simulink model "HW7"  (R2024a)
settings: Solver=ode45  StartTime=0.0  StopTime=300  RelTol=1e-6  EnableMultiTasking=on
values from neighbouring files (symbols this model uses):
  A = [eye(3) -sqrt(3)/3*[1 1 1]' ]*Iwi    [set_up_HW7.m]    (also in setupConstantRateSDA.m)
  accelmax = 2/Iwi    (= 0.02)    [set_up_HW7.m]    (also in setupConstantRateSDA.m)
  c = Q(:,2)    [d2q.m]    (also in mbi.m = trace(Id)*.03; set_up_HW7.m = 0.001)
  I = [3000 0 0 ... (first row only)    [Constants_gui.m]    (also in constants.m; mbi.m = [15, .25, .20; set_up_HW7.m = I-Id; setupConstantRateSDA.m)
  Id = eye(3)*trace(I)*.003    [mbi.m]    (also in set_up_HW7.m = eye(3)*100)
  invI = inv(I)    [Constants_gui.m]    (also in constants.m; mbi.m; set_up_HW7.m; setupConstantRateSDA.m)
  invId = inv(Id)    [mbi.m]    (also in set_up_HW7.m)
  Kd = 2*zet*wn*I    [Constants_gui.m]    (also in constants.m = 2 * zet * wn * I; mbi.m = -eye(3)*.00002; set_up_HW7.m = 375000; setupConstantRateSDA.m)
  Kp = 2*wn^2*I    [Constants_gui.m]    (also in constants.m = 2 * wn^2 * I; mbi.m = -eye(3)*5.5; set_up_HW7.m = 300000; setupConstantRateSDA.m)
  pinvA = pinv(A)    [set_up_HW7.m]    (also in setupConstantRateSDA.m)
  q_init = q_init/norm(q_init)    [Constants_gui.m]    (also in constants.m = [-0.5 -0.5 -0.5 0.5]; mbi.m = [0 0 0 1]'; set_up_HW7.m = [0 0 0 1]'; setupConstantRateSDA.m)
  wbn_init = pi/30*[0 0 0]'    [Constants_gui.m]    (also in constants.m = pi/180 * [0.1; 0.2; 0.15]; mbi.m = [0 0 0]'; set_up_HW7.m = pi/30*[0 0 .01]'; setupConstantRateSDA.m)
  wdn_init = wbn_init    [mbi.m]    (also in set_up_HW7.m)
  wmax = 150/Iwi    (= 1.5)    [set_up_HW7.m]    (also in setupConstantRateSDA.m)
  ww0 = [0 0 0 0].'    [set_up_HW7.m]    (also in setupConstantRateSDA.m)
settings Model: Creator=Mason  LastModifiedBy=Spencer
settings SolverCC: AlgebraicLoopSolver=TrustRegion
settings DataIOCC: LimitDataPoints=on  SaveFormat=Array  SignalLoggingSaveFormat=ModelDataLogs  ReturnWorkspaceOutputs=off
settings OptimizationCC: ExpressionDepthLimit=2147483647  InitFltsAndDblsToZero=on  LifeSpan=inf
settings DebuggingCC: SaveWithParameterizedLinksMsg=none  UnderspecifiedInitializationDetection=Classic  MergeDetectMultiDrivingBlocksExec=none  SignalResolutionControl=TryResolveAllWithWarning  SolverPrmCheckMsg=warning  MultiTaskDSMMsg=warning  MultiTaskCondExecSysMsg=none  FcnCallInpInsideContextMsg=warning  UnconnectedInputMsg=warning  UnconnectedOutputMsg=warning  UnconnectedLineMsg=warning  StateNameClashWarn=warning  SFUnexpectedBacktrackingDiag=warning  SFNoUnconditionalDefaultTransitionDiag=warning  SFExecutionAtInitializationDiag=none  ArithmeticOperatorsInVariantConditions=warning
settings HardwareCC: ProdBitPerPointer=32  ProdBitPerSizeT=32  ProdBitPerPtrDiffT=32  ProdLargestAtomicFloat=None  ProdIntDivRoundTo=Undefined  ProdEndianess=Unspecified  ProdWordSize=32  ProdHWDeviceType=32-bit Generic
settings ModelReferenceCC: EnableRefExpFcnMdlSchedulingChecks=on  PropagateSignalLabelsOutOfModel=off
settings SFSimCC: SimUseLocalCustomCode=off  CustomCodeUndefinedFunction=UseInterfaceOnly
settings RTWCC: RTWUseLocalCustomCode=off  GPUComputeCapability=3.5  DLArmComputeVersion=19.05
settings CodeAppCC: StateflowObjectComments=on
settings GRTTargetCC: TargetFcnLib=ansi_tfl_tmw.mat  TargetLangStandard=C89/C90 (ANSI)  CombineOutputUpdateFcns=off  GRTInterface=on
settings ConfigComp: CovMetricSettings=dw  CovSaveCumulativeToWorkspaceVar=on  CovSaveSingleToWorkspaceVar=on  CovExternalEMLEnable=off

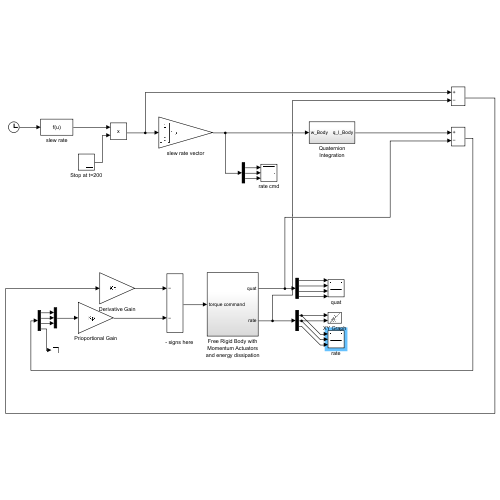
[thumbnail: Simulink's stored preview of the top-level diagram]
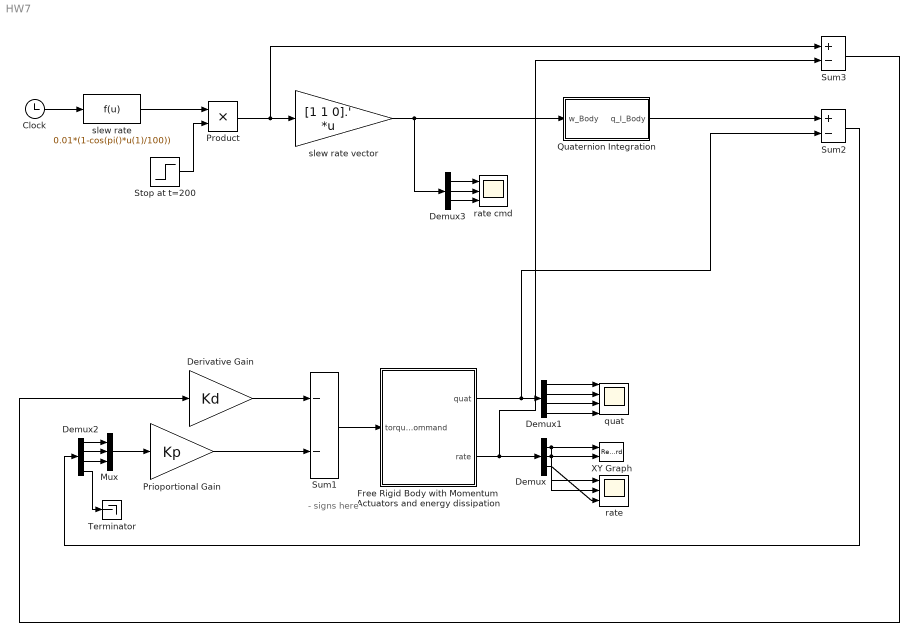
== system HW7 ==
  note: - signs here
  Clock : Clock
  Demux : Demux  Outputs=3
  Demux1 : Demux
  Demux2 : Demux
  Demux3 : Demux  Outputs=3
  Derivative Gain : Gain  Gain=Kd  SaturateOnIntegerOverflow=on  OutDataTypeStr=Inherit: Same as input  ParamDataTypeStr=Inherit: Same as input
  Free Rigid Body with Momentum Actuators and energy dissipation : Subsystem
  Mux : Mux  Inputs=3
  Prioportional Gain : Gain  Gain=Kp  SaturateOnIntegerOverflow=on  OutDataTypeStr=Inherit: Same as input  ParamDataTypeStr=Inherit: Same as input
  Product : Product  InputSameDT=on  SaturateOnIntegerOverflow=on  OutDataTypeStr=Inherit: Same as first input
  Quaternion Integration : Subsystem
  Stop at t=200 : Step  Time=200  Before=1  After=0  SampleTime=0
  Sum1 : Sum  Inputs=--  InputSameDT=on  SaturateOnIntegerOverflow=on  OutDataTypeStr=Inherit: Same as first input
  Sum2 : Sum  Inputs=+-  InputSameDT=on  SaturateOnIntegerOverflow=on  OutDataTypeStr=Inherit: Same as first input
  Sum3 : Sum  Inputs=+-  InputSameDT=on  SaturateOnIntegerOverflow=on  OutDataTypeStr=Inherit: Same as first input
  Terminator : Terminator
  XY Graph : Record  FileSettingsInternal="{\"entries\":[{\"content\":{\"excelSettings\":{\"content\":{},\"type\":\"Streamout.ExcelSettings\"}},\"type\":\"Streamout.FileSettingStorage\",\"uuid\":\"\"}],\"packageUris\":[\"http:\\/\\/schema.mathworks.com\\/mf0\\/streamout_blocks\\/R2020a\"],\"version\":\"1.0\"}"  Layout=[1 1]  SignalsInternal="{\"entries\":[{\"content\":{\"signals\":[{\"content\":{\"blockPath\":[],\"dimensions\":[1],\"domain\":\"\",\"lineColor\":\"#a2142f\",\"plots\":[ 1 ],\"port\":1,\"sid\":[\"\"],\"signalID\":1,\"signalName\":\"Demux:1\"},\"type\":\"RecordBlkView.Signal\",\"uuid\":\"\"},{\"content\":{\"blockPath\":[],\"dimensions\":[1],\"domain\":\"\",\"lineColor\":\"#139fff\",\"plots\":[ 1 ],\"port\":2,\"sid\":[\"\"],\"signalID\":2,\"signalName\":\"Demux:2\"},\"type\":\"RecordBlkView.Signal\",\"uuid\":\"\"}]},\"type\":\"RecordBlkView.InputSignals\",\"uuid\":\"\"}],\"packageUris\":[\"http:\\/\\/schema.mathworks.com\\/mf0\\/streamout_blocks\\/R2020a\"],\"version\":\"1.0\"}"  VisualizationBindings="{\"xyplotplugin\":{\"info\":[{\"series\":[{\"bindingParametersList\":[{\"parameter\":\"X-Axis\",\"signalID\":1,\"signalName\":\"Demux:1\"},{\"parameter\":\"Y-Axis\",\"signalID\":2,\"signalName\":\"Demux:2\"}],\"seriesID\":0}],\"subplotID\":1}]}}"  CompatibilityTag=XY  st=.25
  quat : Scope  NumInputPorts=4
  rate : Scope  NumInputPorts=3
  rate cmd : Scope  NumInputPorts=3
  slew rate : Fcn  Expr=0.01*(1-cos(pi()*u(1)/100))
  slew rate vector : Gain  Gain=[1 1 0].'  Multiplication=Matrix(K*u)  SaturateOnIntegerOverflow=on  OutDataTypeStr=Inherit: Same as input  ParamDataTypeStr=Inherit: Same as input
  wires:
  Demux1/1 -> quat/1
  Demux1/2 -> quat/2
  Demux1/3 -> quat/3
  Demux1/4 -> quat/4
  Demux/1 -> rate/1, XY Graph/1
  Demux/2 -> rate/2, XY Graph/2
  Demux/3 -> rate/3
  Free Rigid Body with Momentum Actuators and energy dissipation/2(rate) -> Sum3/2, Demux/1
  Free Rigid Body with Momentum Actuators and energy dissipation/1(quat) -> Sum2/2, Demux1/1
  Sum1/1 -> Free Rigid Body with Momentum Actuators and energy dissipation/1(torque command)
  Mux/1 -> Prioportional Gain/1
  Derivative Gain/1 -> Sum1/1
  Demux2/2 -> Mux/2
  Demux2/1 -> Mux/1
  Demux2/3 -> Mux/3
  Demux2/4 -> Terminator/1
  Prioportional Gain/1 -> Sum1/2
  Clock/1 -> slew rate/1
  slew rate vector/1 -> Quaternion Integration/1(w_Body), Demux3/1
  Quaternion Integration/1(q_I_Body) -> Sum2/1
  Sum2/1 -> Demux2/1
  Sum3/1 -> Derivative Gain/1
  slew rate/1 -> Product/1
  Stop at t=200/1 -> Product/2
  Product/1 -> Sum3/1, slew rate vector/1
  Demux3/1 -> rate cmd/1
  Demux3/2 -> rate cmd/2
  Demux3/3 -> rate cmd/3

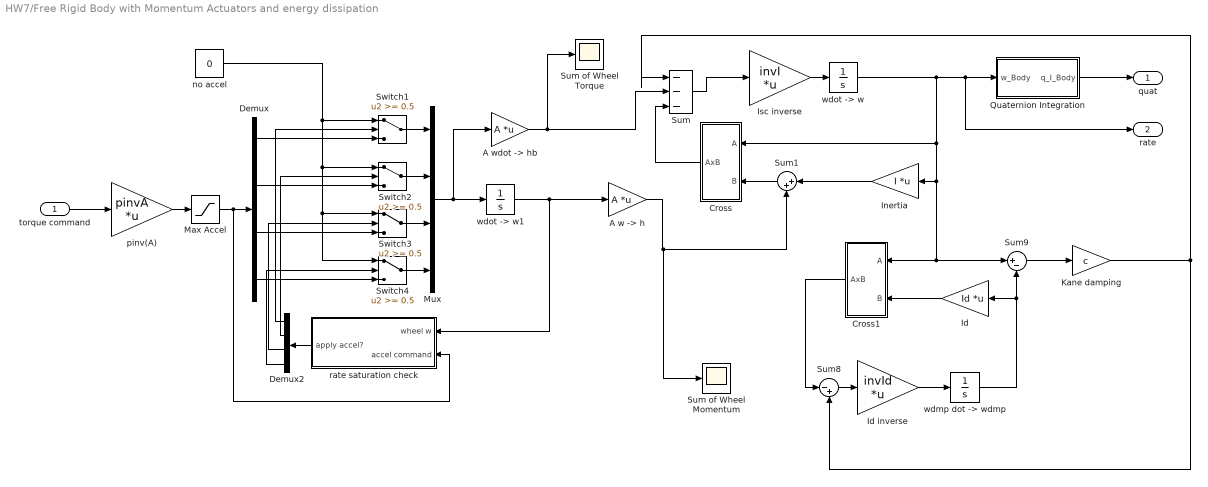
== system HW7/Free Rigid Body with Momentum Actuators and energy dissipation ==
  torque command : Inport
  "A w -> h" : Gain  Gain=A  Multiplication=Matrix(K*u)  SaturateOnIntegerOverflow=on  OutDataTypeStr=Inherit: Same as input  ParamDataTypeStr=Inherit: Same as input
  "A wdot -> hb" : Gain  Gain=A  Multiplication=Matrix(K*u)  SaturateOnIntegerOverflow=on  OutDataTypeStr=Inherit: Same as input  ParamDataTypeStr=Inherit: Same as input
  Cross : Subsystem
  Cross1 : Subsystem
  Demux : Demux
      settings: DisplayOption=none
  Demux2 : Demux
      settings: DisplayOption=none
  Id : Gain  Gain=Id  Multiplication=Matrix(K*u)  SaturateOnIntegerOverflow=on  OutDataTypeStr=Inherit: Same as input  ParamDataTypeStr=Inherit: Same as input
  Id inverse : Gain  Gain=invId  Multiplication=Matrix(K*u)  SaturateOnIntegerOverflow=on  OutDataTypeStr=Inherit: Same as input  ParamDataTypeStr=Inherit: Same as input
  Inertia : Gain  Gain=I  Multiplication=Matrix(K*u)  SaturateOnIntegerOverflow=on  OutDataTypeStr=Inherit: Same as input  ParamDataTypeStr=Inherit: Same as input
  Isc inverse : Gain  Gain=invI  Multiplication=Matrix(K*u)  SaturateOnIntegerOverflow=on  OutDataTypeStr=Inherit: Same as input  ParamDataTypeStr=Inherit: Same as input
  Kane damping : Gain  Gain=c  SaturateOnIntegerOverflow=on  OutDataTypeStr=Inherit: Same as input  ParamDataTypeStr=Inherit: Same as input
  Max Accel : Saturate  UpperLimit=accelmax  LowerLimit=-accelmax
  Mux : Mux
  Quaternion Integration : Subsystem
  Sum : Sum  Inputs=|---  InputSameDT=on  SaturateOnIntegerOverflow=on  OutDataTypeStr=Inherit: Same as first input
  Sum of Wheel Momentum : Scope
  Sum of Wheel Torque : Scope
  Sum1 : Sum  Inputs=|++  InputSameDT=on  SaturateOnIntegerOverflow=on  OutDataTypeStr=Inherit: Same as first input
  Sum8 : Sum  Inputs=|-+  InputSameDT=on  SaturateOnIntegerOverflow=on  OutDataTypeStr=Inherit: Same as first input
  Sum9 : Sum  Inputs=|+-  InputSameDT=on  SaturateOnIntegerOverflow=on  OutDataTypeStr=Inherit: Same as first input
  Switch{1..4} (4 alike) : Switch  Threshold=0.5
  no accel : Constant  Value=0
  pinv(A) : Gain  Gain=pinvA  Multiplication=Matrix(K*u)  SaturateOnIntegerOverflow=on  OutDataTypeStr=Inherit: Same as input  ParamDataTypeStr=Inherit: Same as input
  rate saturation check : Subsystem
  "wdmp dot -> wdmp" : Integrator  InitialCondition=wdn_init
  "wdot -> w" : Integrator  InitialCondition=wbn_init
  "wdot -> w1" : Integrator  InitialCondition=ww0
  quat : Outport
  rate : Outport  Port=2
  wires:
  Isc inverse/1 -> "wdot -> w"/1
  Sum9/1 -> Kane damping/1
  Sum8/1 -> Id inverse/1
  Id/1 -> Cross1/2(B)
  "wdmp dot -> wdmp"/1 -> Id/1, Sum9/2
  Id inverse/1 -> "wdmp dot -> wdmp"/1
  "wdot -> w"/1 -> rate/1, Quaternion Integration/1(w_Body), Sum9/1, Cross1/1(A), Inertia/1, Cross/1(A)
  Sum/1 -> Isc inverse/1
  Cross/1(AxB) -> Sum/3
  Max Accel/1 -> Demux/1, rate saturation check/2(accel command)
  Demux2/1 -> Switch1/2
  Demux2/3 -> Switch3/2
  no accel/1 -> Switch1/1, Switch4/1, Switch3/1, Switch2/1
  pinv(A)/1 -> Max Accel/1
  Demux2/4 -> Switch4/2
  "A wdot -> hb"/1 -> Sum of Wheel Torque/1, Sum/2
  "A w -> h"/1 -> Sum of Wheel Momentum/1, Sum1/2
  Inertia/1 -> Sum1/1
  Sum1/1 -> Cross/2(B)
  Mux/1 -> "wdot -> w1"/1, "A wdot -> hb"/1
  torque command/1 -> pinv(A)/1
  "wdot -> w1"/1 -> "A w -> h"/1, rate saturation check/1(wheel w)
  Quaternion Integration/1(q_I_Body) -> quat/1
  Kane damping/1 -> Sum8/2, Sum/1
  Cross1/1(AxB) -> Sum8/1
  Switch1/1 -> Mux/1
  Switch2/1 -> Mux/2
  Switch3/1 -> Mux/3
  Switch4/1 -> Mux/4
  Demux/1 -> Switch1/3
  Demux/2 -> Switch2/3
  Demux/3 -> Switch3/3
  Demux/4 -> Switch4/3
  rate saturation check/1(apply accel?) -> Demux2/1
  Demux2/2 -> Switch2/2

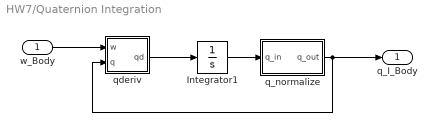
== system HW7/Quaternion Integration ==
  w_Body : Inport
  Integrator1 : Integrator  InitialCondition=q_init
  q_normalize : Subsystem
  qderiv : Subsystem
  q_I_Body : Outport
  wires:
  w_Body/1 -> qderiv/1(w)
  q_normalize/1(q_out) -> qderiv/2(q), q_I_Body/1
  Integrator1/1 -> q_normalize/1(q_in)
  qderiv/1(qd) -> Integrator1/1

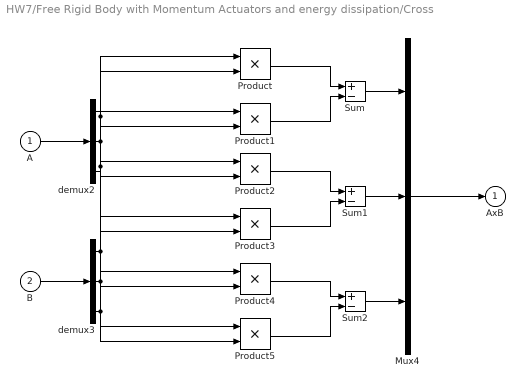
== system HW7/Free Rigid Body with Momentum Actuators and energy dissipation/Cross ==
  A : Inport
  B : Inport  Port=2
  Mux4 : Mux  Inputs=3
  Product{,1..5} (6 alike) : Product  InputSameDT=on  SaturateOnIntegerOverflow=on  OutDataTypeStr=Inherit: Same as first input
  Sum : Sum  Inputs=+-  InputSameDT=on  SaturateOnIntegerOverflow=on  OutDataTypeStr=Inherit: Same as first input
  Sum1 : Sum  Inputs=+-  InputSameDT=on  SaturateOnIntegerOverflow=on  OutDataTypeStr=Inherit: Same as first input
  Sum2 : Sum  Inputs=+-  InputSameDT=on  SaturateOnIntegerOverflow=on  OutDataTypeStr=Inherit: Same as first input
  demux2 : Demux  Outputs=3
      settings: DisplayOption=none
  demux3 : Demux  Outputs=3
      settings: DisplayOption=none
  AxB : Outport  InitialOutput=0
  wires:
  A/1 -> demux2/1
  B/1 -> demux3/1
  demux2/3 -> Product1/1, Product2/1
  demux3/3 -> Product/2, Product3/2
  demux2/1 -> Product3/1, Product4/1
  demux3/2 -> Product1/2, Product4/2
  demux2/2 -> Product/1, Product5/1
  demux3/1 -> Product2/2, Product5/2
  Product/1 -> Sum/1
  Product1/1 -> Sum/2
  Product2/1 -> Sum1/1
  Product3/1 -> Sum1/2
  Product4/1 -> Sum2/1
  Product5/1 -> Sum2/2
  Sum/1 -> Mux4/1
  Sum1/1 -> Mux4/2
  Sum2/1 -> Mux4/3
  Mux4/1 -> AxB/1

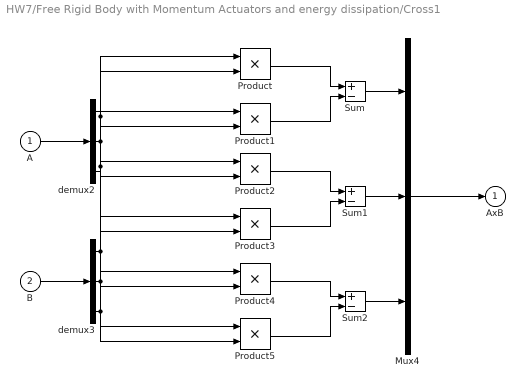
== system HW7/Free Rigid Body with Momentum Actuators and energy dissipation/Cross1 ==
  A : Inport
  B : Inport  Port=2
  Mux4 : Mux  Inputs=3
  Product{,1..5} (6 alike) : Product  InputSameDT=on  SaturateOnIntegerOverflow=on  OutDataTypeStr=Inherit: Same as first input
  Sum : Sum  Inputs=+-  InputSameDT=on  SaturateOnIntegerOverflow=on  OutDataTypeStr=Inherit: Same as first input
  Sum1 : Sum  Inputs=+-  InputSameDT=on  SaturateOnIntegerOverflow=on  OutDataTypeStr=Inherit: Same as first input
  Sum2 : Sum  Inputs=+-  InputSameDT=on  SaturateOnIntegerOverflow=on  OutDataTypeStr=Inherit: Same as first input
  demux2 : Demux  Outputs=3
      settings: DisplayOption=none
  demux3 : Demux  Outputs=3
      settings: DisplayOption=none
  AxB : Outport  InitialOutput=0
  wires:
  A/1 -> demux2/1
  B/1 -> demux3/1
  demux2/3 -> Product1/1, Product2/1
  demux3/3 -> Product/2, Product3/2
  demux2/1 -> Product3/1, Product4/1
  demux3/2 -> Product1/2, Product4/2
  demux2/2 -> Product/1, Product5/1
  demux3/1 -> Product2/2, Product5/2
  Product/1 -> Sum/1
  Product1/1 -> Sum/2
  Product2/1 -> Sum1/1
  Product3/1 -> Sum1/2
  Product4/1 -> Sum2/1
  Product5/1 -> Sum2/2
  Sum/1 -> Mux4/1
  Sum1/1 -> Mux4/2
  Sum2/1 -> Mux4/3
  Mux4/1 -> AxB/1

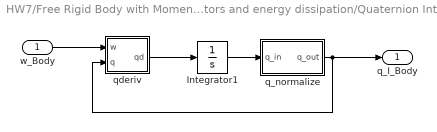
== system HW7/Free Rigid Body with Momentum Actuators and energy dissipation/Quaternion Integration ==
  w_Body : Inport
  Integrator1 : Integrator  InitialCondition=q_init
  q_normalize : Subsystem
  qderiv : Subsystem
  q_I_Body : Outport
  wires:
  w_Body/1 -> qderiv/1(w)
  q_normalize/1(q_out) -> qderiv/2(q), q_I_Body/1
  Integrator1/1 -> q_normalize/1(q_in)
  qderiv/1(qd) -> Integrator1/1

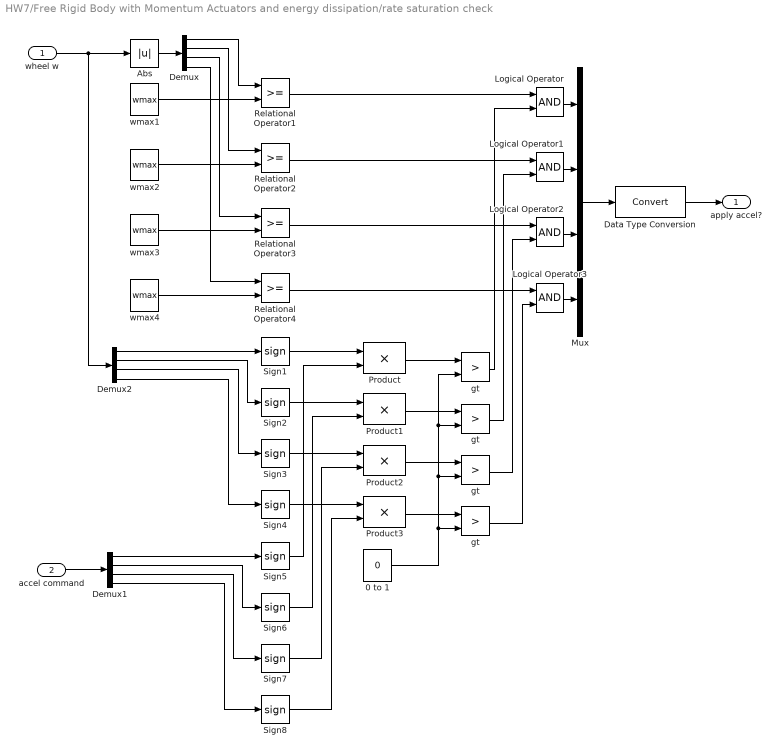
== system HW7/Free Rigid Body with Momentum Actuators and energy dissipation/rate saturation check ==
  wheel w : Inport
  accel command : Inport  Port=2
  0 to 1 : Constant  Value=0  VectorParams1D=off
  Abs : Abs
  Data Type Conversion : DataTypeConversion  SaturateOnIntegerOverflow=off  RndMeth=Floor
  Demux : Demux
      settings: DisplayOption=none
  Demux1 : Demux
      settings: DisplayOption=none
  Demux2 : Demux
      settings: DisplayOption=none
  Logical Operator{,1..3} (4 alike) : Logic
  Mux : Mux
  Product{,1..3} (4 alike) : Product  InputSameDT=on  SaturateOnIntegerOverflow=on  OutDataTypeStr=Inherit: Same as first input
  Relational Operator{1..4} (4 alike) : RelationalOperator
  Sign{1..8} (8 alike) : Signum
  gt : RelationalOperator  Operator=>
  "gt " : RelationalOperator  Operator=>
  "gt  " : RelationalOperator  Operator=>
  "gt   " : RelationalOperator  Operator=>
  wmax{1..4} (4 alike) : Constant  Value=wmax  VectorParams1D=off
  apply accel? : Outport
  wires:
  Abs/1 -> Demux/1
  Demux/1 -> Relational Operator1/1
  Demux/2 -> Relational Operator2/1
  Demux/3 -> Relational Operator3/1
  wmax1/1 -> Relational Operator1/2
  wmax2/1 -> Relational Operator2/2
  wmax3/1 -> Relational Operator3/2
  wheel w/1 -> Abs/1, Demux2/1
  Mux/1 -> Data Type Conversion/1
  accel command/1 -> Demux1/1
  Demux1/2 -> Sign6/1
  Demux1/3 -> Sign7/1
  Sign1/1 -> Product/1
  Sign5/1 -> Product/2
  Sign2/1 -> Product1/1
  Sign6/1 -> Product1/2
  Sign3/1 -> Product2/1
  Sign7/1 -> Product2/2
  Product/1 -> gt/1
  Product1/1 -> "gt "/1
  Product2/1 -> "gt  "/1
  Logical Operator/1 -> Mux/1
  Logical Operator1/1 -> Mux/2
  Logical Operator2/1 -> Mux/3
  Relational Operator1/1 -> Logical Operator/1
  Relational Operator2/1 -> Logical Operator1/1
  Relational Operator3/1 -> Logical Operator2/1
  gt/1 -> Logical Operator/2
  "gt "/1 -> Logical Operator1/2
  "gt  "/1 -> Logical Operator2/2
  Demux2/1 -> Sign1/1
  Demux2/2 -> Sign2/1
  Demux2/3 -> Sign3/1
  Logical Operator3/1 -> Mux/4
  wmax4/1 -> Relational Operator4/2
  Demux/4 -> Relational Operator4/1
  Relational Operator4/1 -> Logical Operator3/1
  0 to 1/1 -> "gt   "/2, "gt  "/2, "gt "/2, gt/2
  Product3/1 -> "gt   "/1
  "gt   "/1 -> Logical Operator3/2
  Demux2/4 -> Sign4/1
  Sign4/1 -> Product3/1
  Sign8/1 -> Product3/2
  Demux1/4 -> Sign8/1
  Demux1/1 -> Sign5/1
  Data Type Conversion/1 -> apply accel?/1

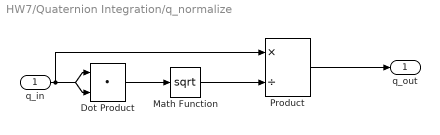
== system HW7/Quaternion Integration/q_normalize ==
  q_in : Inport  PortDimensions=4
  Dot Product : DotProduct  OutDataTypeStr=Inherit: Inherit via internal rule
  Math Function : Math  Operator=sqrt  SignedPower=on
  Product : Product  Inputs=*/  InputSameDT=on  SaturateOnIntegerOverflow=on  OutDataTypeStr=Inherit: Same as first input
  q_out : Outport
  wires:
  Product/1 -> q_out/1
  Math Function/1 -> Product/2
  Dot Product/1 -> Math Function/1
  q_in/1 -> Product/1, Dot Product/2, Dot Product/1

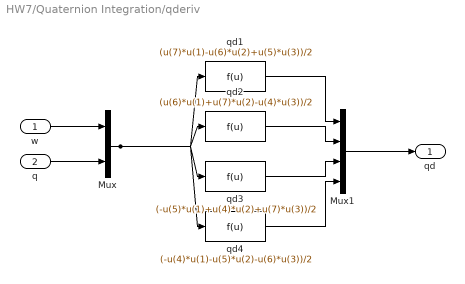
== system HW7/Quaternion Integration/qderiv ==
  w : Inport
  q : Inport  Port=2
  Mux : Mux  Inputs=2
  Mux1 : Mux
  qd1 : Fcn  Expr=(u(7)*u(1)-u(6)*u(2)+u(5)*u(3))/2
  qd2 : Fcn  Expr=(u(6)*u(1)+u(7)*u(2)-u(4)*u(3))/2
  qd3 : Fcn  Expr=(-u(5)*u(1)+u(4)*u(2)+u(7)*u(3))/2
  qd4 : Fcn  Expr=(-u(4)*u(1)-u(5)*u(2)-u(6)*u(3))/2
  qd : Outport
  wires:
  Mux1/1 -> qd/1
  qd4/1 -> Mux1/4
  qd3/1 -> Mux1/3
  qd2/1 -> Mux1/2
  qd1/1 -> Mux1/1
  Mux/1 -> qd4/1, qd3/1, qd2/1, qd1/1
  q/1 -> Mux/2
  w/1 -> Mux/1

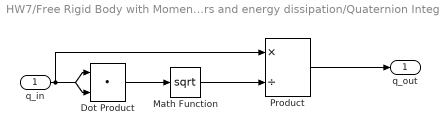
== system HW7/Free Rigid Body with Momentum Actuators and energy dissipation/Quaternion Integration/q_normalize ==
  q_in : Inport  PortDimensions=4
  Dot Product : DotProduct  OutDataTypeStr=Inherit: Inherit via internal rule
  Math Function : Math  Operator=sqrt  SignedPower=on
  Product : Product  Inputs=*/  InputSameDT=on  SaturateOnIntegerOverflow=on  OutDataTypeStr=Inherit: Same as first input
  q_out : Outport
  wires:
  Product/1 -> q_out/1
  Math Function/1 -> Product/2
  Dot Product/1 -> Math Function/1
  q_in/1 -> Product/1, Dot Product/2, Dot Product/1

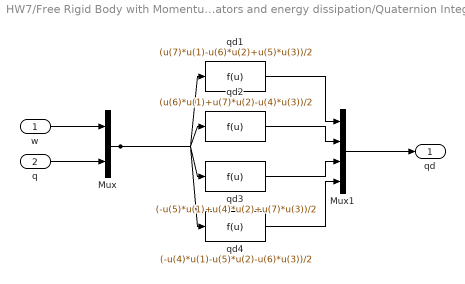
== system HW7/Free Rigid Body with Momentum Actuators and energy dissipation/Quaternion Integration/qderiv ==
  w : Inport
  q : Inport  Port=2
  Mux : Mux  Inputs=2
  Mux1 : Mux
  qd1 : Fcn  Expr=(u(7)*u(1)-u(6)*u(2)+u(5)*u(3))/2
  qd2 : Fcn  Expr=(u(6)*u(1)+u(7)*u(2)-u(4)*u(3))/2
  qd3 : Fcn  Expr=(-u(5)*u(1)+u(4)*u(2)+u(7)*u(3))/2
  qd4 : Fcn  Expr=(-u(4)*u(1)-u(5)*u(2)-u(6)*u(3))/2
  qd : Outport
  wires:
  Mux1/1 -> qd/1
  qd4/1 -> Mux1/4
  qd3/1 -> Mux1/3
  qd2/1 -> Mux1/2
  qd1/1 -> Mux1/1
  Mux/1 -> qd4/1, qd3/1, qd2/1, qd1/1
  q/1 -> Mux/2
  w/1 -> Mux/1
